simulink model "untitled1"  (R2023a)
settings: Solver=VariableStepAuto  StartTime=0.0  StopTime=0.01  RelTol=1e-4
values from neighbouring files (symbols this model uses):
  C = 1e-5    (= 1e-05)    [Problem2_lab03.m]    (also in script1.m)
  R = 2000    [Problem2_lab03.m]    (also in script1.m)
undefined symbols (not defined in the file or in its folder): L
settings Model: Creator=mcconncm  LastModifiedBy=mcconncm

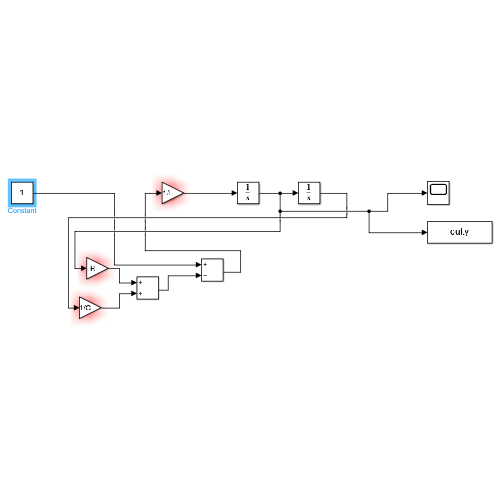
[thumbnail: Simulink's stored preview of the top-level diagram]
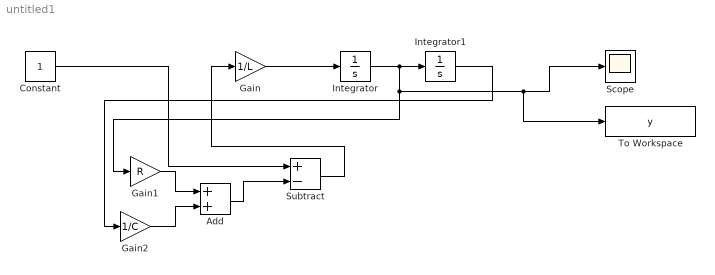
== system untitled1 ==
  Add : Sum
  Constant : Constant
  Gain : Gain  Gain=1/L
  Gain1 : Gain  Gain=R
  Gain2 : Gain  Gain=1/C
  Integrator : Integrator
  Integrator1 : Integrator
  Scope : Scope
  Subtract : Sum  Inputs=+-
  To Workspace : ToWorkspace  VariableName=y  SampleTime=-1
  wires:
  Integrator/1 -> To Workspace/1, Scope/1, Gain1/1, Integrator1/1
  Integrator1/1 -> Gain2/1
  Gain/1 -> Integrator/1
  Gain1/1 -> Add/1
  Gain2/1 -> Add/2
  Add/1 -> Subtract/2
  Constant/1 -> Subtract/1
  Subtract/1 -> Gain/1
